simulink model "preg1"  (R2021a)
settings: Solver=VariableStepAuto  StartTime=0.0  StopTime=10.0  RelTol=1e-3
settings Model: Creator=Felipe  LastModifiedBy=Felipe

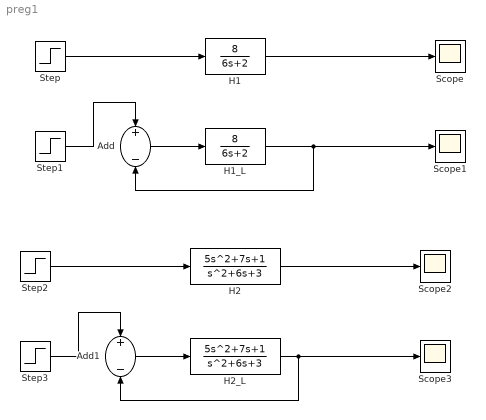
== system preg1 ==
  Add : Sum  Inputs=+-
  Add1 : Sum  Inputs=+-
  H1 : TransferFcn  Numerator=[8]  Denominator=[6 2]
  H1_L : TransferFcn  Numerator=[8]  Denominator=[6 2]
  H2 : TransferFcn  Numerator=[5 7 1]  Denominator=[1 6 3]
  H2_L : TransferFcn  Numerator=[5 7 1]  Denominator=[1 6 3]
  Scope{,1..3} (4 alike) : Scope
  Step{,1..3} (4 alike) : Step  SampleTime=0
  wires:
  Step/1 -> H1/1
  H1/1 -> Scope/1
  Add/1 -> H1_L/1
  H1_L/1 -> Add/2, Scope1/1
  Step1/1 -> Add/1
  Add1/1 -> H2_L/1
  H2_L/1 -> Add1/2, Scope3/1
  H2/1 -> Scope2/1
  Step2/1 -> H2/1
  Step3/1 -> Add1/1
